simulink model "Ej4"  (R2018a)
settings: Solver=ode45  StartTime=0.0  StopTime=30  RelTol=1e-6  AbsTol=1e-6
values from neighbouring files (symbols this model uses):
  a = 200    [Ej1_params.m]    (also in Ej2_params.m; Ej3_params.m; Ej4_params.m)
  b = 10000    [Ej1_params.m]    (also in Ej2_params.m; Ej3_params.m; Ej4_params.m)
  g = 9.82    [Ej1_params.m]    (also in Ej2_params.m; Ej3_params.m; Ej4_params.m)
  kd = double(subs(kd_solu, [m_s, a_s, b_s, p_place_s], [m, a, b, p_place]))    [Ej4_params.m]
  ki = .1    (= 0.1)    [Ej3_params.m]    (also in Ej4_params.m = double(subs(ki_solu, [m_s, a_s, b_s, p_place_s], [m, a, b, p)
  kp = 1    [Ej3_params.m]    (also in Ej4_params.m = double(subs(kp_solu, [m_s, a_s, b_s, p_place_s], [m, a, b, p)
  m = 1500    [Ej1_params.m]    (also in Ej2_params.m = 1000; Ej3_params.m = 1000; Ej4_params.m = 1000)
libraries: simulink_extras x2
settings Model: Creator=joses  LastModifiedBy=joses

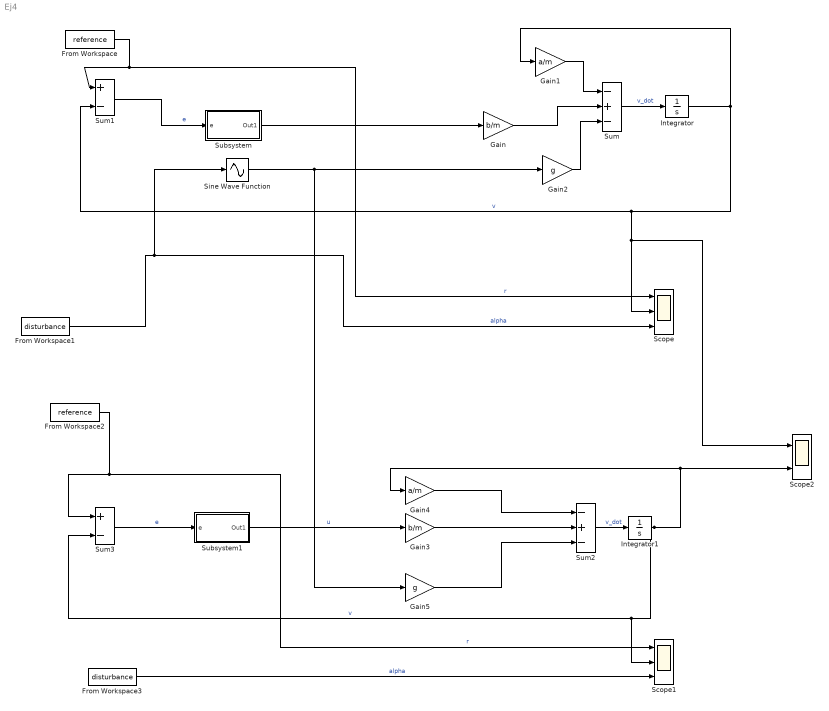
== system Ej4 ==
  From Workspace : FromWorkspace  VariableName=reference  SampleTime=.01
  From Workspace1 : FromWorkspace  VariableName=disturbance  SampleTime=.01
  From Workspace2 : FromWorkspace  VariableName=reference  SampleTime=.01
  From Workspace3 : FromWorkspace  VariableName=disturbance  SampleTime=.01
  Gain : Gain  Gain=b/m
  Gain1 : Gain  Gain=a/m
  Gain2 : Gain  Gain=g
  Gain3 : Gain  Gain=b/m
  Gain4 : Gain  Gain=a/m
  Gain5 : Gain  Gain=g
  Integrator : Integrator
  Integrator1 : Integrator
  Scope : Scope  NumInputPorts=3
  Scope1 : Scope  NumInputPorts=3
  Scope2 : Scope  NumInputPorts=2
  Sine Wave Function : Sin  TimeSource=Use external signal  SampleTime=0
  Subsystem : Subsystem
  Subsystem1 : Subsystem
  Sum : Sum  Inputs=-+-
  Sum1 : Sum  Inputs=+-
  Sum2 : Sum  Inputs=-+-
  Sum3 : Sum  Inputs=+-
  wires:
  Sum/1 -> Integrator/1  "v_dot"
  Gain/1 -> Sum/2
  Gain1/1 -> Sum/1
  Integrator/1 -> Gain1/1, Sum1/2, Scope2/1, Scope/2  "v"
  From Workspace/1 -> Scope/1, Sum1/1  "r"
  From Workspace1/1 -> Sine Wave Function/1, Scope/3  "alpha"
  Gain2/1 -> Sum/3
  From Workspace2/1 -> Sum3/1, Scope1/1  "r"
  From Workspace3/1 -> Scope1/3  "alpha"
  Sum3/1 -> Subsystem1/1(e)  "e"
  Gain5/1 -> Sum2/3
  Sine Wave Function/1 -> Gain5/1, Gain2/1
  Gain4/1 -> Sum2/1
  Sum2/1 -> Integrator1/1  "v_dot"
  Integrator1/1 -> Scope2/2, Gain4/1, Sum3/2, Scope1/2  "v"
  Subsystem1/1(Out1) -> Gain3/1  "u"
  Gain3/1 -> Sum2/2
  Sum1/1 -> Subsystem/1(e)  "e"
  Subsystem/1(Out1) -> Gain/1

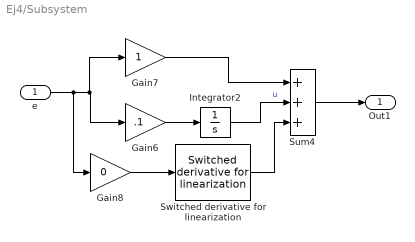
== system Ej4/Subsystem ==
  e : Inport
  Gain6 : Gain  Gain=.1
  Gain7 : Gain
  Gain8 : Gain  Gain=0
  Integrator2 : Integrator
  Sum4 : Sum  Inputs=+++
  Switched derivative for linearization : simulink_extras/Linearization/Switched derivative for linearization  switchVal=0  derivConst=1000
      settings: SourceProductName=Simulink  SourceProductBaseCode=SL
  Out1 : Outport
  wires:
  Gain8/1 -> Switched derivative for linearization/1
  e/1 -> Gain8/1, Gain7/1, Gain6/1
  Integrator2/1 -> Sum4/2  "u"
  Gain7/1 -> Sum4/1
  Gain6/1 -> Integrator2/1
  Sum4/1 -> Out1/1
  Switched derivative for linearization/1 -> Sum4/3

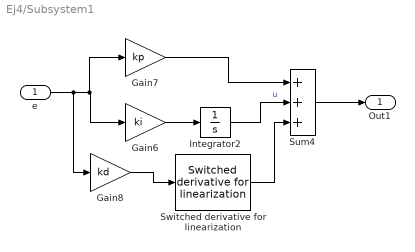
== system Ej4/Subsystem1 ==
  e : Inport
  Gain6 : Gain  Gain=ki
  Gain7 : Gain  Gain=kp
  Gain8 : Gain  Gain=kd
  Integrator2 : Integrator
  Sum4 : Sum  Inputs=+++
  Switched derivative for linearization : simulink_extras/Linearization/Switched derivative for linearization  switchVal=0  derivConst=1000
      settings: SourceProductName=Simulink  SourceProductBaseCode=SL
  Out1 : Outport
  wires:
  Gain8/1 -> Switched derivative for linearization/1
  Switched derivative for linearization/1 -> Sum4/3
  e/1 -> Gain8/1, Gain7/1, Gain6/1
  Integrator2/1 -> Sum4/2  "u"
  Gain7/1 -> Sum4/1
  Gain6/1 -> Integrator2/1
  Sum4/1 -> Out1/1
